simulink model "two_virtual_wheel_discrete"  (Simulink 7.8)
settings: Solver=FixedStepDiscrete  SolverMode=MultiTasking  StartTime=0.0  StopTime=tfinal  RelTol=1e-3
values from neighbouring files (symbols this model uses):
  b1 = T1*k1    (= 0.15)    [two_virtual_wheel_params.m]    (also in two_virtual_wheels.m)
  b2 = T2*k2    (= 0.015)    [two_virtual_wheel_params.m]    (also in two_virtual_wheels.m)
  Jw1 = .5*1.5/4    (= 0.1875)    [two_virtual_wheel_params.m]    (also in two_virtual_wheels.m)
  Jw2 = .5*.015/4    (= 0.001875)    [two_virtual_wheel_params.m]    (also in two_virtual_wheels.m)
  k1 = .5*15    (= 7.5)    [two_virtual_wheel_params.m]    (also in two_virtual_wheels.m)
  k2 = .5*15    (= 7.5)    [two_virtual_wheel_params.m]    (also in two_virtual_wheels.m)
  step_time = 1    [two_virtual_wheel_params.m]    (also in two_virtual_wheels.m)
  T1 = 1/50    (= 0.02)    [two_virtual_wheel_params.m]    (also in two_virtual_wheels.m)
  T2 = 1/500    (= 0.002)    [two_virtual_wheel_params.m]    (also in two_virtual_wheels.m)
  Theta_z_0 = 45    [two_virtual_wheel_params.m]    (also in two_virtual_wheels.m)
undefined symbols (not defined in the file or in its folder): DiscIntNeverNeededParam
settings Model: Creator=Embed_Sys_course  LastModifiedBy=Embed_Sys_course  ExtModeTrigMode=oneshot  ExtModeArmWhenConnect=off
settings DataIOCC: LimitDataPoints=off  SignalLoggingName=sigsOut
settings OptimizationCC: BooleanDataType=off  InitFltsAndDblsToZero=on
settings DebuggingCC: SaveWithParameterizedLinksMsg=none  SignalResolutionControl=TryResolveAllWithWarning  SolverPrmCheckMsg=none  MultiTaskDSMMsg=warning  MultiTaskCondExecSysMsg=none  FcnCallInpInsideContextMsg=Use local settings  StrictBusMsg=None
settings HardwareCC: TargetUnknown=on
settings RTWCC: IncludeERTFirstTime=on
settings GRTTargetCC: TargetFcnLib=ansi_tfl_tmw.mat

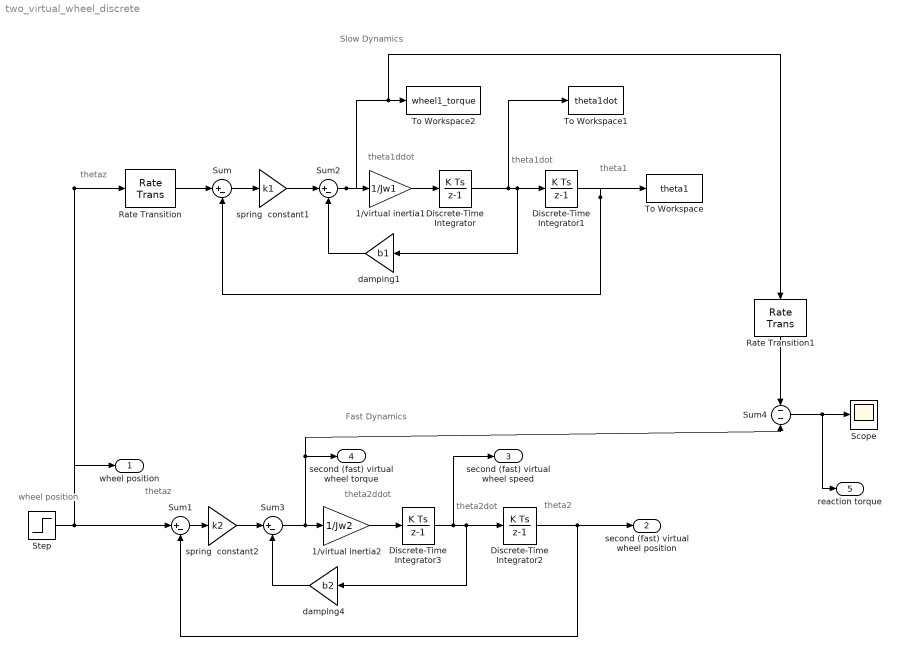
== system two_virtual_wheel_discrete ==
  note: theta1
  note: theta1dot
  note: theta1ddot
  note: thetaz
  note: theta2
  note: theta2dot
  note: theta2ddot
  note: thetaz
  note: wheel position
  note: Fast Dynamics
  note: Slow Dynamics
  1/virtual inertia1 : Gain  Gain=1/Jw1  SaturateOnIntegerOverflow=on  OutDataTypeStr=Inherit: Same as input  ParamDataTypeStr=Inherit: Same as input
  1/virtual inertia2 : Gain  Gain=1/Jw2  SaturateOnIntegerOverflow=on  OutDataTypeStr=Inherit: Same as input  ParamDataTypeStr=Inherit: Same as input
  Discrete-Time Integrator : DiscreteIntegrator  SampleTime=T1  ICPrevOutput=DiscIntNeverNeededParam  ICPrevScaledInput=DiscIntNeverNeededParam
  Discrete-Time Integrator1 : DiscreteIntegrator  SampleTime=T1  ICPrevOutput=DiscIntNeverNeededParam  ICPrevScaledInput=DiscIntNeverNeededParam
  Discrete-Time Integrator2 : DiscreteIntegrator  SampleTime=T2  ICPrevOutput=DiscIntNeverNeededParam  ICPrevScaledInput=DiscIntNeverNeededParam
  Discrete-Time Integrator3 : DiscreteIntegrator  SampleTime=T2  ICPrevOutput=DiscIntNeverNeededParam  ICPrevScaledInput=DiscIntNeverNeededParam
  Rate Transition : RateTransition
  Rate Transition1 : RateTransition
  Scope : Scope
  Step : Step  Time=step_time  After=Theta_z_0  SampleTime=T2
  Sum{,1..3} (4 alike) : Sum  Inputs=|+-  SaturateOnIntegerOverflow=on  InputSameDT=on  OutDataTypeStr=Inherit: Same as first input
  Sum4 : Sum  Inputs=-|-  SaturateOnIntegerOverflow=on  InputSameDT=on  OutDataTypeStr=Inherit: Same as first input
  To Workspace : ToWorkspace  VariableName=theta1  SampleTime=-1  SaveFormat=Structure With Time
  To Workspace1 : ToWorkspace  VariableName=theta1dot  SampleTime=-1  SaveFormat=Structure With Time
  To Workspace2 : ToWorkspace  VariableName=wheel1_torque  SampleTime=-1  SaveFormat=Structure With Time
  damping1 : Gain  Gain=b1  SaturateOnIntegerOverflow=on  OutDataTypeStr=Inherit: Same as input  ParamDataTypeStr=Inherit: Same as input
  damping4 : Gain  Gain=b2  SaturateOnIntegerOverflow=on  OutDataTypeStr=Inherit: Same as input  ParamDataTypeStr=Inherit: Same as input
  spring  constant1 : Gain  Gain=k1  SaturateOnIntegerOverflow=on  OutDataTypeStr=Inherit: Same as input  ParamDataTypeStr=Inherit: Same as input
  spring  constant2 : Gain  Gain=k2  SaturateOnIntegerOverflow=on  OutDataTypeStr=Inherit: Same as input  ParamDataTypeStr=Inherit: Same as input
  wheel position : Outport
  second (fast) virtual wheel position : Outport  Port=2
  second (fast) virtual wheel speed : Outport  Port=3
  second (fast) virtual wheel torque : Outport  Port=4
  reaction torque : Outport  Port=5
  wires:
  Discrete-Time Integrator1/1 -> Sum/2, To Workspace/1
  Sum/1 -> spring  constant1/1
  Step/1 -> wheel position/1, Rate Transition/1, Sum1/1
  1/virtual inertia1/1 -> Discrete-Time Integrator/1
  Discrete-Time Integrator/1 -> Discrete-Time Integrator1/1, damping1/1, To Workspace1/1
  Discrete-Time Integrator2/1 -> Sum1/2, second (fast) virtual wheel position/1
  Sum1/1 -> spring  constant2/1
  1/virtual inertia2/1 -> Discrete-Time Integrator3/1
  Discrete-Time Integrator3/1 -> Discrete-Time Integrator2/1, damping4/1, second (fast) virtual wheel speed/1
  spring  constant1/1 -> Sum2/1
  Sum2/1 -> 1/virtual inertia1/1, Rate Transition1/1, To Workspace2/1
  damping1/1 -> Sum2/2
  Sum3/1 -> 1/virtual inertia2/1, second (fast) virtual wheel torque/1, Sum4/2
  damping4/1 -> Sum3/2
  spring  constant2/1 -> Sum3/1
  Sum4/1 -> reaction torque/1, Scope/1
  Rate Transition1/1 -> Sum4/1
  Rate Transition/1 -> Sum/1
